simulink model "Test_Bit_Multiplexer_2_to_1"  (Simulink 8.1)
settings: Solver=ode45  StartTime=0.0  StopTime=len  RelTol=1e-3
libraries: commutil2 x2, Bit_Multiplexers_Lib x1
settings Model: Creator=N  LastModifiedBy=uzivatel
settings DataIOCC: LimitDataPoints=off  SignalLoggingSaveFormat=Dataset
settings OptimizationCC: ExpressionDepthLimit=128
settings DebuggingCC: UnderspecifiedInitializationDetection=Simplified  MergeDetectMultiDrivingBlocksExec=error  SolverPrmCheckMsg=none  FcnCallInpInsideContextMsg=EnableAllAsError  FrameProcessingCompatibilityMsg=error  StateNameClashWarn=none
settings HardwareCC: ProdBitPerPointer=64  ProdLargestAtomicFloat=Float  ProdIntDivRoundTo=Zero  ProdEndianess=LittleEndian  ProdHWDeviceType=Intel->x86-64 (Windows64)
settings ModelReferenceCC: PropagateSignalLabelsOutOfModel=on
settings GRTTargetCC: CodeReplacementLibrary=None  CombineOutputUpdateFcns=on  CPPClassGenCompliant=on  GRTInterface=off

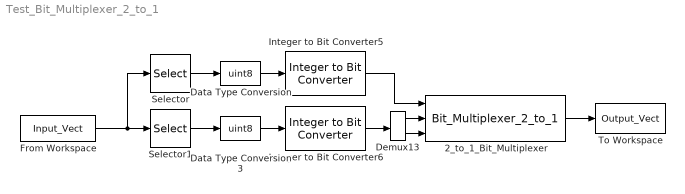
== system Test_Bit_Multiplexer_2_to_1 ==
  2_to_1_Bit_Multiplexer : Bit_Multiplexers_Lib/Bit_Multiplexers_Lib/Bit_Multiplexer_2_to_1
  Data Type Conversion : DataTypeConversion  OutDataTypeStr=uint8
  Data Type Conversion3 : DataTypeConversion  OutDataTypeStr=uint8
  Demux13 : Demux  Outputs=2
  From Workspace : FromWorkspace  VariableName=Input_Vect  SampleTime=1  Interpolate=off  OutputAfterFinalValue=Holding final value
  Integer to Bit Converter5 : commutil2/Integer to Bit Converter  nbits=1  signedInputValues=Unsigned  bitOrder=MSB first  outDtype=uint8
  Integer to Bit Converter6 : commutil2/Integer to Bit Converter  nbits=2  signedInputValues=Unsigned  bitOrder=MSB first  outDtype=uint8
  Selector : Selector  IndexMode=Zero-based  InputPortWidth=2  SampleTime=1  IndexOptions=Index vector (dialog)  Indices=0  OutputSizes=1
  Selector1 : Selector  IndexMode=Zero-based  InputPortWidth=2  IndexOptions=Index vector (dialog)  Indices=1  OutputSizes=1
  To Workspace : ToWorkspace  VariableName=Output_Vect  SampleTime=1
  wires:
  Demux13/2 -> 2_to_1_Bit_Multiplexer/3
  Demux13/1 -> 2_to_1_Bit_Multiplexer/2
  From Workspace/1 -> Selector/1, Selector1/1
  Integer to Bit Converter5/1 -> 2_to_1_Bit_Multiplexer/1
  Integer to Bit Converter6/1 -> Demux13/1
  Selector/1 -> Data Type Conversion/1
  Selector1/1 -> Data Type Conversion3/1
  Data Type Conversion/1 -> Integer to Bit Converter5/1
  Data Type Conversion3/1 -> Integer to Bit Converter6/1
  2_to_1_Bit_Multiplexer/1 -> To Workspace/1
